simulink model "FIR_FILTER"  (R2020b)
settings: Solver=VariableStepAuto  StartTime=0.0  StopTime=10  RelTol=1e-3
model workspace (MAT data in the model file):
  Sig = Simulink.Signal
  Sig.DataType = 'auto'
  Sig.Dimensions = -1
  Sig.DimensionsMode = 'auto'
  Sig.Complexity = 'auto'
  Sig.SampleTime = -1
  Sig.SamplingMode = 'auto'
undefined symbols (not defined in the file): a1, a2, a3, a4
settings Model: DataDictionary=fir_filter_data_Dictionary.sldd  Creator=intel  LastModifiedBy=intel
settings DataIOCC: SaveOutput=off  SaveTime=off

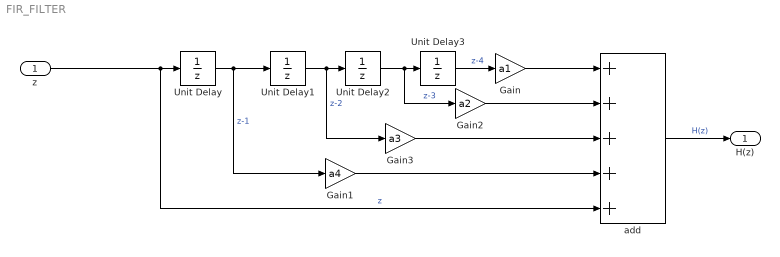
== system FIR_FILTER ==
  z : Inport  OutDataTypeStr=double  PortDimensions=1  SampleTime=0
  Gain : Gain  Gain=a1
  Gain1 : Gain  Gain=a4
  Gain2 : Gain  Gain=a2
  Gain3 : Gain  Gain=a3
  Unit Delay{,1..3} (4 alike) : UnitDelay  SampleTime=-1  HasFrameUpgradeWarning=on
  add : Sum  Inputs=+++++
  H(z) : Outport  OutDataTypeStr=double  PortDimensions=1  SampleTime=0
  wires:
  Unit Delay1/1 -> Unit Delay2/1, Gain3/1  "z-2"
  Gain3/1 -> add/3
  z/1 -> Unit Delay/1, add/5  "z"
  Unit Delay2/1 -> Unit Delay3/1, Gain2/1  "z-3"
  Unit Delay/1 -> Unit Delay1/1, Gain1/1  "z-1"
  Gain/1 -> add/1
  Unit Delay3/1 -> Gain/1  "z-4"
  Gain1/1 -> add/4
  Gain2/1 -> add/2
  add/1 -> H(z)/1  "H(z)"
